simulink library "MATLAB_Function_lib"  (R2017b)
settings: Solver=VariableStepAuto  StartTime=0.0  StopTime=10.0  RelTol=1e-3
undefined symbols (not defined in the file or in its folder): Newton, Raphson
libraries: simulink x1
(part 2 of 3)

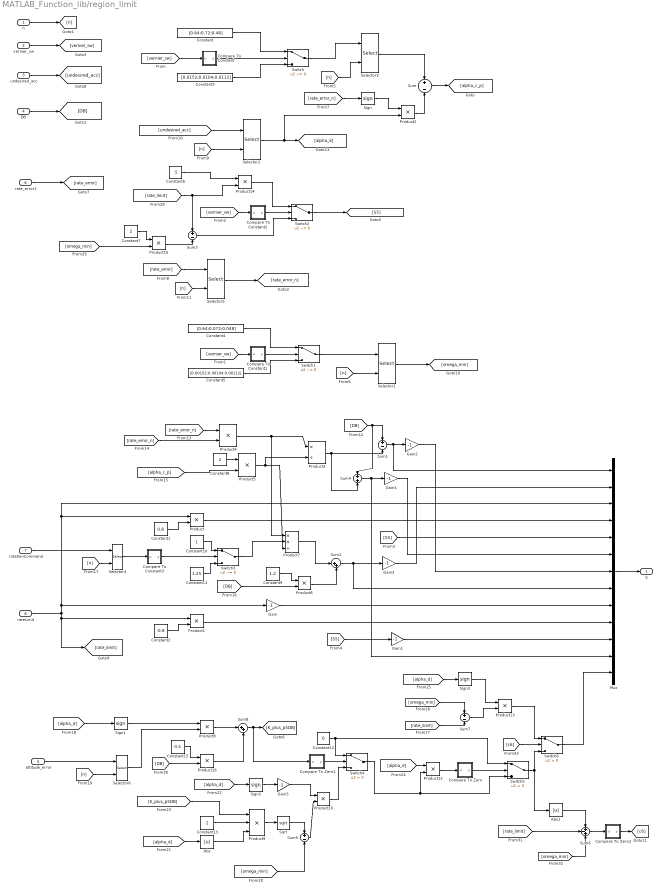
== system MATLAB_Function_lib/region_limit ==
  n : Inport
  vernier_sw : Inport  Port=2
  undesired_acc : Inport  Port=3
  DB : Inport  Port=4
  attitude_error : Inport  Port=5
  rate_error1 : Inport  Port=6
  rotationCommand : Inport  Port=7
  rateLimit : Inport  Port=8
  Abs : Abs
  Abs1 : Abs
  Compare To Constant : Subsystem  mask(Compare To Constant){relop===, const=1, OutDataTypeStr=boolean, ZeroCross=on}
      mask prompts: relop "Simulink:masks:Operator_MP"; const "Simulink:masks:ConstantValue_MP"; OutDataTypeStr "Simulink:masks:OutputDataType_MP"; ZeroCross "Simulink:masks:EnableZerocrossingDetection_MP"
      mask help: Simulink:masks:CompareToConstant_MD
      mask init: same as MATLAB_Function_lib/phase_plane/Compare To Constant
      mask TypeOptions relop: == | ~= | < | <= | >= | >
      mask TypeOptions OutDataTypeStr: Simulink:masks:uint8 | Simulink:masks:boolean
      mask Callback ZeroCross: sl('zeroCrossEnable', gcbh);
      mask Display: disp(str)
  Compare To Constant1 : Subsystem  mask(Compare To Constant){relop===, const=1, OutDataTypeStr=boolean, ZeroCross=on}
      mask prompts: relop "Simulink:masks:Operator_MP"; const "Simulink:masks:ConstantValue_MP"; OutDataTypeStr "Simulink:masks:OutputDataType_MP"; ZeroCross "Simulink:masks:EnableZerocrossingDetection_MP"
      mask help: Simulink:masks:CompareToConstant_MD
      mask init: same as MATLAB_Function_lib/phase_plane/Compare To Constant
      mask TypeOptions relop: == | ~= | < | <= | >= | >
      mask TypeOptions OutDataTypeStr: Simulink:masks:uint8 | Simulink:masks:boolean
      mask Callback ZeroCross: sl('zeroCrossEnable', gcbh);
      mask Display: disp(str)
  Compare To Constant2 : Subsystem  mask(Compare To Constant){relop===, const=0, OutDataTypeStr=boolean, ZeroCross=on}
      mask prompts: relop "Simulink:masks:Operator_MP"; const "Simulink:masks:ConstantValue_MP"; OutDataTypeStr "Simulink:masks:OutputDataType_MP"; ZeroCross "Simulink:masks:EnableZerocrossingDetection_MP"
      mask help: Simulink:masks:CompareToConstant_MD
      mask init: same as MATLAB_Function_lib/phase_plane/Compare To Constant
      mask TypeOptions relop: == | ~= | < | <= | >= | >
      mask TypeOptions OutDataTypeStr: Simulink:masks:uint8 | Simulink:masks:boolean
      mask Callback ZeroCross: sl('zeroCrossEnable', gcbh);
      mask Display: disp(str)
  Compare To Constant3 : Subsystem  mask(Compare To Constant){relop===, const=1, OutDataTypeStr=boolean, ZeroCross=on}
      mask prompts: relop "Simulink:masks:Operator_MP"; const "Simulink:masks:ConstantValue_MP"; OutDataTypeStr "Simulink:masks:OutputDataType_MP"; ZeroCross "Simulink:masks:EnableZerocrossingDetection_MP"
      mask help: Simulink:masks:CompareToConstant_MD
      mask init: same as MATLAB_Function_lib/phase_plane/Compare To Constant
      mask TypeOptions relop: == | ~= | < | <= | >= | >
      mask TypeOptions OutDataTypeStr: Simulink:masks:uint8 | Simulink:masks:boolean
      mask Callback ZeroCross: sl('zeroCrossEnable', gcbh);
      mask Display: disp(str)
  Compare To Zero : Subsystem  mask(Compare To Zero){relop=>, OutDataTypeStr=boolean, ZeroCross=on}
      mask prompts: relop "Simulink:masks:Operator_MP"; OutDataTypeStr "Simulink:masks:OutputDataType_MP"; ZeroCross "Simulink:masks:EnableZerocrossingDetection_MP"
      mask help: Simulink:masks:CompareToZero_MD
      mask init: same as MATLAB_Function_lib/affectation_region/Compare To Zero2
      mask TypeOptions relop: == | ~= | < | <= | >= | >
      mask TypeOptions OutDataTypeStr: Simulink:masks:uint8 | Simulink:masks:boolean
      mask Callback ZeroCross: sl('zeroCrossEnable', gcbh);
      mask Display: disp([relop,' 0'])
  Compare To Zero1 : Subsystem  mask(Compare To Zero){relop=<=, OutDataTypeStr=boolean, ZeroCross=on}
      mask prompts: relop "Simulink:masks:Operator_MP"; OutDataTypeStr "Simulink:masks:OutputDataType_MP"; ZeroCross "Simulink:masks:EnableZerocrossingDetection_MP"
      mask help: Simulink:masks:CompareToZero_MD
      mask init: same as MATLAB_Function_lib/affectation_region/Compare To Zero2
      mask TypeOptions relop: == | ~= | < | <= | >= | >
      mask TypeOptions OutDataTypeStr: Simulink:masks:uint8 | Simulink:masks:boolean
      mask Callback ZeroCross: sl('zeroCrossEnable', gcbh);
      mask Display: disp([relop,' 0'])
  Compare To Zero2 : Subsystem  mask(Compare To Zero){relop=>, OutDataTypeStr=boolean, ZeroCross=on}
      mask prompts: relop "Simulink:masks:Operator_MP"; OutDataTypeStr "Simulink:masks:OutputDataType_MP"; ZeroCross "Simulink:masks:EnableZerocrossingDetection_MP"
      mask help: Simulink:masks:CompareToZero_MD
      mask init: same as MATLAB_Function_lib/affectation_region/Compare To Zero2
      mask TypeOptions relop: == | ~= | < | <= | >= | >
      mask TypeOptions OutDataTypeStr: Simulink:masks:uint8 | Simulink:masks:boolean
      mask Callback ZeroCross: sl('zeroCrossEnable', gcbh);
      mask Display: disp([relop,' 0'])
  Constant : Constant  Value=[0.64;0.72;0.48]
  Constant1 : Constant  Value=0.8
  Constant10 : Constant
  Constant11 : Constant  Value=1.25
  Constant12 : Constant  Value=0
  Constant13 : Constant  Value=2
  Constant15 : Constant  Value=0.5
  Constant2 : Constant  Value=-0.8
  Constant3 : Constant  Value=[0.0152;0.0104;0.0112]
  Constant4 : Constant  Value=[0.64;0.072;0.048]
  Constant5 : Constant  Value=[0.00152;0.00104;0.00112]
  Constant6 : Constant  Value=.5
  Constant7 : Constant  Value=2
  Constant8 : Constant  Value=2
  Constant9 : Constant  Value=1.2
  Gain{,1..5} (6 alike) : Gain  Gain=-1
  Mux : Mux  Inputs=13
  Product{,1..2,6,8,10,12..16} (11 alike) : Product
  Product3 : Product  Inputs=*/
  Product4 : Product  Inputs=**
  Product5 : Product  Inputs=**
  Product7 : Product  Inputs=**/
  Product9 : Product  Inputs=3
  Selector{1..6} (6 alike) : Selector  InputPortWidth=3  IndexOptions=Index vector (port)  Indices=[1 3]  OutputSizes=1
  Sign{,1..3} (4 alike) : Signum
  Sqrt : Sqrt  SaturateOnIntegerOverflow=on
  Sum{,1,3,5,7} (5 alike) : Sum  Inputs=+-
  Sum2 : Sum  Inputs=|++
  Sum4 : Sum
  Sum6 : Sum  Inputs=+-+
  Sum8 : Sum  Inputs=|++
  Switch{,1..3} (4 alike) : Switch  Criteria=u2 ~= 0
  Switch4 : Switch  Criteria=u2 > Threshold
  Switch5 : Switch  Criteria=u2 > Threshold
  Switch6 : Switch  Criteria=u2 > Threshold
  S : Outport  PortDimensions=13
  wires:
  attitude_error/1 -> Selector6/1
  undesired_acc/1 -> [undesired_acc]
  vernier_sw/1 -> [vernier_sw]
  n/1 -> [n]
  DB/1 -> [DB]
  rate_error1/1 -> [rate_error]
  Mux/1 -> S/1
  Product/1 -> Mux/4
  Constant1/1 -> Product/2
  Product1/1 -> Mux/10
  rateLimit/1 -> Product1/1, [rate_limit], Mux/3, Product/1, Gain/1
  Constant2/1 -> Product1/2
  Gain/1 -> Mux/9
  [vernier_sw] -> Compare To Constant/1(u)
  Compare To Constant/1(y) -> Switch/2
  Constant/1 -> Switch/1
  Constant3/1 -> Switch/3
  Constant4/1 -> Switch1/1
  [vernier_sw] -> Compare To Constant1/1(u)
  Constant5/1 -> Switch1/3
  Compare To Constant1/1(y) -> Switch1/2
  Product14/1 -> Switch2/1
  [vernier_sw] -> Compare To Constant2/1(u)
  Sum3/1 -> Switch2/3
  Compare To Constant2/1(y) -> Switch2/2
  Switch2/1 -> [S5]
  [S5] -> Mux/5
  [S5] -> Gain1/1
  Gain1/1 -> Mux/11
  [n] -> Selector3/2
  Selector3/1 -> Sum/1
  Switch/1 -> Selector3/1
  Selector1/1 -> [omega_min]
  [n] -> Selector1/2
  Switch1/1 -> Selector1/1
  Selector2/1 -> Product2/2, [alpha_d]
  [n] -> Selector2/2
  [undesired_acc] -> Selector2/1
  Product2/1 -> Sum/2
  Sum/1 -> [alpha_c_p]
  [rate_error_n] -> Sign/1
  Sign/1 -> Product2/1
  [rate_error] -> Selector5/1
  Selector5/1 -> [rate_error_n]
  [n] -> Selector5/2
  [DB] -> Sum4/1, Sum1/1
  Product3/1 -> Sum4/2, Sum1/2
  [rate_error_n] -> Product4/1
  [rate_error_n] -> Product4/2
  Product4/1 -> Product7/1, Product3/1
  Product5/1 -> Product7/3, Product3/2
  Constant8/1 -> Product5/1
  [alpha_c_p] -> Product5/2
  Sum1/1 -> Mux/1, Gain2/1
  Gain2/1 -> Mux/7
  Product6/1 -> Sum2/2
  Constant9/1 -> Product6/1
  [DB] -> Product6/2
  Sum2/1 -> Mux/8, Gain3/1
  Gain3/1 -> Mux/2
  Product7/1 -> Sum2/1
  Switch3/1 -> Product7/2
  Constant10/1 -> Switch3/1
  Constant11/1 -> Switch3/3
  [n] -> Selector4/2
  rotationCommand/1 -> Selector4/1
  Compare To Constant3/1(y) -> Switch3/2
  Selector4/1 -> Compare To Constant3/1(u)
  Sum4/1 -> Gain4/1, Mux/12
  Gain4/1 -> Mux/6
  Sign1/1 -> Product8/1
  [alpha_d] -> Sign1/1
  Selector6/1 -> Product8/2
  [n] -> Selector6/2
  Product8/1 -> Sum8/1
  Constant12/1 -> Switch5/1, Switch4/1
  [omega_min] -> Sum5/2
  [alpha_d] -> Abs/1
  Abs/1 -> Product9/3
  Constant13/1 -> Product9/2
  Product9/1 -> Sqrt/1
  Sqrt/1 -> Sum5/1
  Sum5/1 -> Product10/2
  [alpha_d] -> Sign2/1
  Sign2/1 -> Gain5/1
  Gain5/1 -> Product10/1
  Product10/1 -> Switch4/3
  [K_plus_p5DB] -> Product9/1
  Product12/1 -> Compare To Zero/1(u)
  Compare To Zero/1(y) -> Switch5/2
  [alpha_d] -> Product12/1
  Switch4/1 -> Switch5/3, Product12/2
  [alpha_d] -> Sign3/1
  Sign3/1 -> Product13/1
  Product13/1 -> Switch6/1
  Switch5/1 -> Abs1/1, Switch6/3
  [omega_min] -> Sum7/1
  [rate_limit] -> Sum7/2
  Sum7/1 -> Product13/2
  Switch6/1 -> Mux/13
  Constant6/1 -> Product14/1
  [rate_limit] -> Sum3/1, Product14/2
  Product15/1 -> Sum3/2
  Constant7/1 -> Product15/1
  [omega_min] -> Product15/2
  Constant15/1 -> Product16/1
  [DB] -> Product16/2
  Product16/1 -> Sum8/2
  Sum8/1 -> Compare To Zero1/1(u), [K_plus_p5DB]
  Compare To Zero1/1(y) -> Switch4/2
  Compare To Zero2/1(y) -> [c6]
  Sum6/1 -> Compare To Zero2/1(u)
  Abs1/1 -> Sum6/1
  [rate_limit] -> Sum6/2
  [omega_min] -> Sum6/3
  [c6] -> Switch6/2

== system MATLAB_Function_lib/vernier_jet_logic ==
  Constant : Constant  Value=zeros(6,1)
  Out1 : Outport
  wires:
  Constant/1 -> Out1/1

== system MATLAB_Function_lib/Direction Cosine Matrix to Quaternions/Negative Trace ==
  DCM : Inport
  Action Port : ActionPort  PropagateVarSize=During execution  ActionType=else
  Find Maximum Diagonal Value : If  NumInputs=3  IfExpression=((u2 > u1) & (u2 > u3))  ElseIfExpressions=u3 > u1
  Maximum Value at DCM(1,1) : Subsystem
  Maximum Value at DCM(2,2) : Subsystem
  Maximum Value at DCM(3,3) : Subsystem
  Merge1 : Merge  Inputs=3
  diag(DCM) : Subsystem
  qw qx qy qz : Outport
  wires:
  Find Maximum Diagonal Value/2 -> Maximum Value at DCM(3,3)/Action
  DCM/1 -> diag(DCM)/1(DCM), Maximum Value at DCM(2,2)/1(DCM), Maximum Value at DCM(1,1)/1(DCM), Maximum Value at DCM(3,3)/1(DCM)
  diag(DCM)/1(u(1)) -> Find Maximum Diagonal Value/1
  Merge1/1 -> qw qx qy qz/1
  Maximum Value at DCM(1,1)/1(qw qx qy qz) -> Merge1/3
  diag(DCM)/3(u(9)) -> Find Maximum Diagonal Value/3
  Maximum Value at DCM(2,2)/1(qw qx qy qz) -> Merge1/1
  Find Maximum Diagonal Value/3 -> Maximum Value at DCM(1,1)/Action
  Maximum Value at DCM(3,3)/1(qw qx qy qz) -> Merge1/2
  diag(DCM)/2(u(5)) -> Find Maximum Diagonal Value/2
  Find Maximum Diagonal Value/1 -> Maximum Value at DCM(2,2)/Action

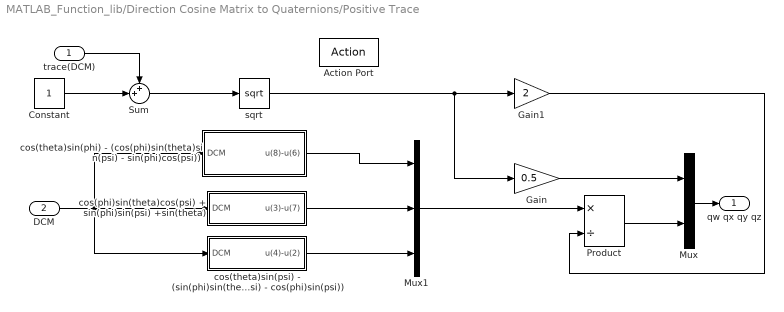
== system MATLAB_Function_lib/Direction Cosine Matrix to Quaternions/Positive Trace ==
  trace(DCM) : Inport
  DCM : Inport  Port=2
  Action Port : ActionPort  PropagateVarSize=During execution  ActionType=then
  Constant : Constant  OutDataTypeStr=Inherit: Inherit via back propagation
  Gain : Gain  Gain=0.5  OutDataTypeStr=Inherit: Inherit via back propagation  SaturateOnIntegerOverflow=on  ParamDataTypeStr=Inherit: Same as input
  Gain1 : Gain  Gain=2  OutDataTypeStr=Inherit: Inherit via back propagation  SaturateOnIntegerOverflow=on  ParamDataTypeStr=Inherit: Same as input
  Mux : Mux  Inputs=2
  Mux1 : Mux  Inputs=3
  Product : Product  Inputs=*/  SaturateOnIntegerOverflow=on  InputSameDT=on  OutDataTypeStr=Inherit: Same as first input
  Sum : Sum  Inputs=++|  SaturateOnIntegerOverflow=on  InputSameDT=on  OutDataTypeStr=Inherit: Same as first input
  cos(phi)sin(theta)cos(psi) + sin(phi)sin(psi) +sin(theta) : Subsystem
  cos(theta)sin(phi) - (cos(phi)sin(theta)sin(psi) - sin(phi)cos(psi)) : Subsystem
  cos(theta)sin(psi) - (sin(phi)sin(theta)cos(psi) - cos(phi)sin(psi)) : Subsystem
  sqrt : Sqrt  AlgorithmType=Newton-Raphson  SaturateOnIntegerOverflow=on
  qw qx qy qz : Outport
  wires:
  sqrt/1 -> Gain/1, Gain1/1
  trace(DCM)/1 -> Sum/1
  Mux1/1 -> Product/1
  Constant/1 -> Sum/2
  Sum/1 -> sqrt/1
  Gain1/1 -> Product/2
  Gain/1 -> Mux/1
  Mux/1 -> qw qx qy qz/1
  Product/1 -> Mux/2
  cos(phi)sin(theta)cos(psi) + sin(phi)sin(psi) +sin(theta)/1(u(3)-u(7)) -> Mux1/2
  cos(theta)sin(psi) - (sin(phi)sin(theta)cos(psi) - cos(phi)sin(psi))/1(u(4)-u(2)) -> Mux1/3
  cos(theta)sin(phi) - (cos(phi)sin(theta)sin(psi) - sin(phi)cos(psi))/1(u(8)-u(6)) -> Mux1/1
  DCM/1 -> cos(theta)sin(phi) - (cos(phi)sin(theta)sin(psi) - sin(phi)cos(psi))/1(DCM), cos(phi)sin(theta)cos(psi) + sin(phi)sin(psi) +sin(theta)/1(DCM), cos(theta)sin(psi) - (sin(phi)sin(theta)cos(psi) - cos(phi)sin(psi))/1(DCM)

== system MATLAB_Function_lib/Direction Cosine Matrix to Quaternions/trace(DCM) ==
  DCM : Inport
  Add : Sum  Inputs=+
  Selector : Selector  InputPortWidth=9  IndexOptions=Index vector (dialog)  Indices=[1 5 9]  OutputSizes=1
  trace(DCM) : Outport
  wires:
  DCM/1 -> Selector/1
  Selector/1 -> Add/1
  Add/1 -> trace(DCM)/1

== system MATLAB_Function_lib/Quaternion Multiplication/q0 ==
  q : Inport
  r : Inport  Port=2
  Demux : Demux
  Demux1 : Demux
  Product{,1..3} (4 alike) : Product  RndMeth=Zero
  Sum : Sum  Inputs=+---
  q0 : Outport
  wires:
  Product2/1 -> Sum/3
  Sum/1 -> q0/1
  Product3/1 -> Sum/4
  Product1/1 -> Sum/2
  Product/1 -> Sum/1
  Demux/4 -> Product3/1
  Demux1/4 -> Product3/2
  Demux1/3 -> Product2/2
  Demux/3 -> Product2/1
  Demux1/2 -> Product1/2
  Demux/2 -> Product1/1
  Demux1/1 -> Product/2
  Demux/1 -> Product/1
  r/1 -> Demux1/1
  q/1 -> Demux/1

== system MATLAB_Function_lib/Quaternion Multiplication/q1 ==
  q : Inport
  r : Inport  Port=2
  Demux : Demux
  Demux1 : Demux
  Product{,1..3} (4 alike) : Product  RndMeth=Zero
  Sum : Sum  Inputs=+++-
  q1 : Outport
  wires:
  Demux1/3 -> Product3/2
  Demux1/4 -> Product2/2
  Demux1/1 -> Product1/2
  Demux1/2 -> Product/2
  q/1 -> Demux/1
  r/1 -> Demux1/1
  Demux/1 -> Product/1
  Demux/2 -> Product1/1
  Demux/3 -> Product2/1
  Demux/4 -> Product3/1
  Product/1 -> Sum/1
  Product1/1 -> Sum/2
  Product3/1 -> Sum/4
  Sum/1 -> q1/1
  Product2/1 -> Sum/3

== system MATLAB_Function_lib/Quaternion Multiplication/q2 ==
  q : Inport
  r : Inport  Port=2
  Demux : Demux
  Demux1 : Demux
  Product{,1..3} (4 alike) : Product  RndMeth=Zero
  Sum : Sum  Inputs=+-++
  q2 : Outport
  wires:
  Demux1/2 -> Product3/2
  Demux1/1 -> Product2/2
  Demux1/4 -> Product1/2
  Demux1/3 -> Product/2
  Product2/1 -> Sum/3
  Sum/1 -> q2/1
  Product3/1 -> Sum/4
  Product1/1 -> Sum/2
  Product/1 -> Sum/1
  Demux/4 -> Product3/1
  Demux/3 -> Product2/1
  Demux/2 -> Product1/1
  Demux/1 -> Product/1
  r/1 -> Demux1/1
  q/1 -> Demux/1

== system MATLAB_Function_lib/Quaternion Multiplication/q3 ==
  q : Inport
  r : Inport  Port=2
  Demux : Demux
  Demux1 : Demux
  Product{,1..3} (4 alike) : Product  RndMeth=Zero
  Sum : Sum  Inputs=++-+
  q3 : Outport
  wires:
  Demux1/4 -> Product/2
  Demux1/3 -> Product1/2
  Demux1/1 -> Product3/2
  Demux1/2 -> Product2/2
  q/1 -> Demux/1
  r/1 -> Demux1/1
  Demux/1 -> Product/1
  Demux/2 -> Product1/1
  Demux/3 -> Product2/1
  Demux/4 -> Product3/1
  Product/1 -> Sum/1
  Product1/1 -> Sum/2
  Product3/1 -> Sum/4
  Sum/1 -> q3/1
  Product2/1 -> Sum/3

== system MATLAB_Function_lib/Rotation Angles to Direction Cosine Matrix/Create 3x3 Matrix ==
  M11 : Inport  PortDimensions=1
  M12 : Inport  Port=2  PortDimensions=1
  M13 : Inport  Port=3  PortDimensions=1
  M21 : Inport  Port=4  PortDimensions=1
  M22 : Inport  Port=5  PortDimensions=1
  M23 : Inport  Port=6  PortDimensions=1
  M31 : Inport  Port=7  PortDimensions=1
  M32 : Inport  Port=8  PortDimensions=1
  M33 : Inport  Port=9  PortDimensions=1
  Reshape (9) to [3x3] column-major : Reshape  OutputDimensionality=Customize  OutputDimensions=[3,3]
  Vector Concatenate : Concatenate  NumInputs=9
  Matrix : Outport  PortDimensions=[3 3]
  wires:
  M33/1 -> Vector Concatenate/9
  M23/1 -> Vector Concatenate/8
  M13/1 -> Vector Concatenate/7
  M32/1 -> Vector Concatenate/6
  Reshape (9) to [3x3] column-major/1 -> Matrix/1
  M22/1 -> Vector Concatenate/5
  M12/1 -> Vector Concatenate/4
  M31/1 -> Vector Concatenate/3
  M21/1 -> Vector Concatenate/2
  M11/1 -> Vector Concatenate/1
  Vector Concatenate/1 -> Reshape (9) to [3x3] column-major/1

== system MATLAB_Function_lib/affectation_region/Compare To Zero2 ==
  u : Inport
  Compare : RelationalOperator  Operator=>  OutDataTypeStr=boolean  RndMeth=Nearest  InputSameDT=on
  Constant : Constant  DisableCoverage=on  Value=0  OutDataTypeStr=Inherit: Inherit via back propagation  PreserveConstantTs=on
  y : Outport
  wires:
  Constant/1 -> Compare/2
  u/1 -> Compare/1
  Compare/1 -> y/1

== system MATLAB_Function_lib/affectation_region/Compare To Zero20 ==
  u : Inport
  Compare : RelationalOperator  OutDataTypeStr=boolean  RndMeth=Nearest  InputSameDT=on
  Constant : Constant  DisableCoverage=on  Value=0  OutDataTypeStr=Inherit: Inherit via back propagation  PreserveConstantTs=on
  y : Outport
  wires:
  Constant/1 -> Compare/2
  u/1 -> Compare/1
  Compare/1 -> y/1

== system MATLAB_Function_lib/affectation_region/Compare To Zero23 ==
  u : Inport
  Compare : RelationalOperator  OutDataTypeStr=boolean  RndMeth=Nearest  InputSameDT=on
  Constant : Constant  DisableCoverage=on  Value=0  OutDataTypeStr=Inherit: Inherit via back propagation  PreserveConstantTs=on
  y : Outport
  wires:
  Constant/1 -> Compare/2
  u/1 -> Compare/1
  Compare/1 -> y/1

== system MATLAB_Function_lib/affectation_region/Compare To Zero26 ==
  u : Inport
  Compare : RelationalOperator  Operator=<  OutDataTypeStr=boolean  RndMeth=Nearest  InputSameDT=on
  Constant : Constant  DisableCoverage=on  Value=0  OutDataTypeStr=Inherit: Inherit via back propagation  PreserveConstantTs=on
  y : Outport
  wires:
  Constant/1 -> Compare/2
  u/1 -> Compare/1
  Compare/1 -> y/1

== system MATLAB_Function_lib/affectation_region/Compare To Zero39 ==
  u : Inport
  Compare : RelationalOperator  Operator=<=  OutDataTypeStr=boolean  RndMeth=Nearest  InputSameDT=on
  Constant : Constant  DisableCoverage=on  Value=0  OutDataTypeStr=Inherit: Inherit via back propagation  PreserveConstantTs=on
  y : Outport
  wires:
  Constant/1 -> Compare/2
  u/1 -> Compare/1
  Compare/1 -> y/1

== system MATLAB_Function_lib/affectation_region/Compare To Zero42 ==
  u : Inport
  Compare : RelationalOperator  Operator=>  OutDataTypeStr=boolean  RndMeth=Nearest  InputSameDT=on
  Constant : Constant  DisableCoverage=on  Value=0  OutDataTypeStr=Inherit: Inherit via back propagation  PreserveConstantTs=on
  y : Outport
  wires:
  Constant/1 -> Compare/2
  u/1 -> Compare/1
  Compare/1 -> y/1

== system MATLAB_Function_lib/affectation_region/Compare To Zero7 ==
  u : Inport
  Compare : RelationalOperator  Operator=<=  OutDataTypeStr=boolean  RndMeth=Nearest  InputSameDT=on
  Constant : Constant  DisableCoverage=on  Value=0  OutDataTypeStr=Inherit: Inherit via back propagation  PreserveConstantTs=on
  y : Outport
  wires:
  Constant/1 -> Compare/2
  u/1 -> Compare/1
  Compare/1 -> y/1

== system MATLAB_Function_lib/get_delta_omega/For Iterator Subsystem ==
  JetCommand : Inport
  matrix_delta_omega_jet : Inport  Port=2
  Compare To Constant : Subsystem  mask(Compare To Constant){relop===, const=1, OutDataTypeStr=boolean, ZeroCross=on}
      mask prompts: relop "Simulink:masks:Operator_MP"; const "Simulink:masks:ConstantValue_MP"; OutDataTypeStr "Simulink:masks:OutputDataType_MP"; ZeroCross "Simulink:masks:EnableZerocrossingDetection_MP"
      mask help: Simulink:masks:CompareToConstant_MD
      mask init: same as MATLAB_Function_lib/phase_plane/Compare To Constant
      mask TypeOptions relop: == | ~= | < | <= | >= | >
      mask TypeOptions OutDataTypeStr: Simulink:masks:uint8 | Simulink:masks:boolean
      mask Callback ZeroCross: sl('zeroCrossEnable', gcbh);
      mask Display: disp(str)
  For Iterator : ForIterator  ResetStates=reset  IterationLimit=11
  Reshape : Reshape  OutputDimensionality=Column vector (2-D)
  Selector1 : Selector  InputPortWidth=11  IndexOptions=Index vector (port)  Indices=[1 3]  OutputSizes=1
  Selector2 : Selector  NumberOfDimensions=2  InputPortWidth=3  IndexOptions=Index vector (port),Select all  Indices=[1 3],1  OutputSizes=1,1
  Sum : Sum  Inputs=|++
  Switch : Switch  Criteria=u2 ~= 0
  Unit Delay : UnitDelay  InitialCondition=[0; 0; 0]  SampleTime=-1
  Out1 : Outport
  wires:
  matrix_delta_omega_jet/1 -> Selector2/1
  For Iterator/1 -> Selector1/2, Selector2/2
  JetCommand/1 -> Selector1/1
  Selector1/1 -> Compare To Constant/1(u)
  Compare To Constant/1(y) -> Switch/2
  Sum/1 -> Switch/1
  Selector2/1 -> Reshape/1
  Switch/1 -> Unit Delay/1, Out1/1
  Unit Delay/1 -> Sum/2, Switch/3
  Reshape/1 -> Sum/1

== system MATLAB_Function_lib/phase_plane/Compare To Constant ==
  u : Inport
  Compare : RelationalOperator  Operator===  OutDataTypeStr=boolean  RndMeth=Nearest  InputSameDT=on
  Constant : Constant  DisableCoverage=on  Value=const  OutDataTypeStr=Inherit: Inherit via back propagation
  y : Outport
  wires:
  u/1 -> Compare/1
  Constant/1 -> Compare/2
  Compare/1 -> y/1

== system MATLAB_Function_lib/phase_plane/Compare To Constant1 ==
  u : Inport
  Compare : RelationalOperator  Operator===  OutDataTypeStr=boolean  RndMeth=Nearest  InputSameDT=on
  Constant : Constant  DisableCoverage=on  Value=const  OutDataTypeStr=Inherit: Inherit via back propagation
  y : Outport
  wires:
  u/1 -> Compare/1
  Constant/1 -> Compare/2
  Compare/1 -> y/1

== system MATLAB_Function_lib/phase_plane/Compare To Constant2 ==
  u : Inport
  Compare : RelationalOperator  Operator===  OutDataTypeStr=boolean  RndMeth=Nearest  InputSameDT=on
  Constant : Constant  DisableCoverage=on  Value=const  OutDataTypeStr=Inherit: Inherit via back propagation
  y : Outport
  wires:
  u/1 -> Compare/1
  Constant/1 -> Compare/2
  Compare/1 -> y/1

== system MATLAB_Function_lib/phase_plane/Compare To Constant3 ==
  u : Inport
  Compare : RelationalOperator  Operator===  OutDataTypeStr=boolean  RndMeth=Nearest  InputSameDT=on
  Constant : Constant  DisableCoverage=on  Value=const  OutDataTypeStr=Inherit: Inherit via back propagation
  y : Outport
  wires:
  u/1 -> Compare/1
  Constant/1 -> Compare/2
  Compare/1 -> y/1

== system MATLAB_Function_lib/phase_plane/If Action Subsystem ==
  Action Port : ActionPort
  Constant : Constant  Value=-1
  Out1 : Outport
  wires:
  Constant/1 -> Out1/1

== system MATLAB_Function_lib/phase_plane/If Action Subsystem1 ==
  Action Port : ActionPort
  Constant : Constant
  Out1 : Outport
  wires:
  Constant/1 -> Out1/1

== system MATLAB_Function_lib/phase_plane/If Action Subsystem2 ==
  Action Port : ActionPort
  Constant : Constant  Value=0
  Out1 : Outport
  wires:
  Constant/1 -> Out1/1

== system MATLAB_Function_lib/phase_plane/If Action Subsystem3 ==
  we : Inport
  rateLimit : Inport  Port=2
  Action Port : ActionPort
  Constant : Constant  Value=3.2
  Constant1 : Constant  Value=4
  Product : Product  Inputs=**/
  Sum : Sum  Inputs=+-
  Out1 : Outport
  wires:
  Sum/1 -> Out1/1
  Constant/1 -> Sum/1
  Product/1 -> Sum/2
  rateLimit/1 -> Product/3
  we/1 -> Product/2
  Constant1/1 -> Product/1

== system MATLAB_Function_lib/phase_plane/If Action Subsystem4 ==
  we : Inport
  rateLimit : Inport  Port=2
  Action Port : ActionPort
  Constant : Constant  Value=3.2
  Constant1 : Constant  Value=4
  Product : Product  Inputs=**/
  Sum : Sum  Inputs=+-
  Out1 : Outport
  wires:
  Product/1 -> Sum/2
  Constant/1 -> Sum/1
  Constant1/1 -> Product/1
  we/1 -> Product/2
  rateLimit/1 -> Product/3
  Sum/1 -> Out1/1

== system MATLAB_Function_lib/phase_plane/If Action Subsystem5 ==
  forceFire_n : Inport
  S13 : Inport  Port=2
  we : Inport  Port=3
  rateLimit : Inport  Port=4
  Action Port : ActionPort
  Constant : Constant  Value=-1  SampleTime=-1
  Constant1 : Constant  Value=0.8
  Product : Product  Inputs=**/
  Sum : Sum  Inputs=+-
  Sum1 : Sum  Inputs=+-
  Switch : Switch  Criteria=u2 ~= 0
  Out1 : Outport
  wires:
  Switch/1 -> Out1/1
  forceFire_n/1 -> Switch/2
  Constant/1 -> Switch/1
  Product/1 -> Switch/3
  Constant1/1 -> Product/1
  S13/1 -> Sum1/2, Sum/1
  we/1 -> Sum/2
  Sum1/1 -> Product/3
  Sum/1 -> Product/2
  rateLimit/1 -> Sum1/1

== system MATLAB_Function_lib/phase_plane/If Action Subsystem6 ==
  forceFire_n : Inport
  S13 : Inport  Port=2
  we : Inport  Port=3
  rateLimit : Inport  Port=4
  Action Port : ActionPort
  Constant : Constant  SampleTime=-1
  Constant1 : Constant  Value=0.8
  Product : Product  Inputs=**/
  Sum : Sum  Inputs=+-
  Sum1 : Sum
  Switch : Switch  Criteria=u2 ~= 0
  Out1 : Outport
  wires:
  Switch/1 -> Out1/1
  we/1 -> Sum/2
  Constant1/1 -> Product/1
  S13/1 -> Sum1/2, Sum/1
  Sum1/1 -> Product/3
  Product/1 -> Switch/3
  forceFire_n/1 -> Switch/2
  Constant/1 -> Switch/1
  Sum/1 -> Product/2
  rateLimit/1 -> Sum1/1

== system MATLAB_Function_lib/phase_plane/If Action Subsystem7 ==
  S13 : Inport
  we : Inport  Port=2
  rateLimit : Inport  Port=3
  Action Port : ActionPort
  Constant1 : Constant  Value=0.8
  Product : Product  Inputs=3
  Product1 : Product
  Sign : Signum
  Sum : Sum  Inputs=+-
  Sum1 : Sum  Inputs=+-
  Out1 : Outport
  wires:
  we/1 -> Sign/1, Sum/2
  Sum1/1 -> Product/3
  rateLimit/1 -> Sum1/1
  Product/1 -> Out1/1
  Sum/1 -> Product/2
  Constant1/1 -> Product/1
  S13/1 -> Product1/1, Sum/1
  Product1/1 -> Sum1/2
  Sign/1 -> Product1/2

== system MATLAB_Function_lib/phase_plane/If Action Subsystem8 ==
  Action Port : ActionPort  ActionType=else
  Constant3 : Constant  Value=-100
  Out1 : Outport
  wires:
  Constant3/1 -> Out1/1

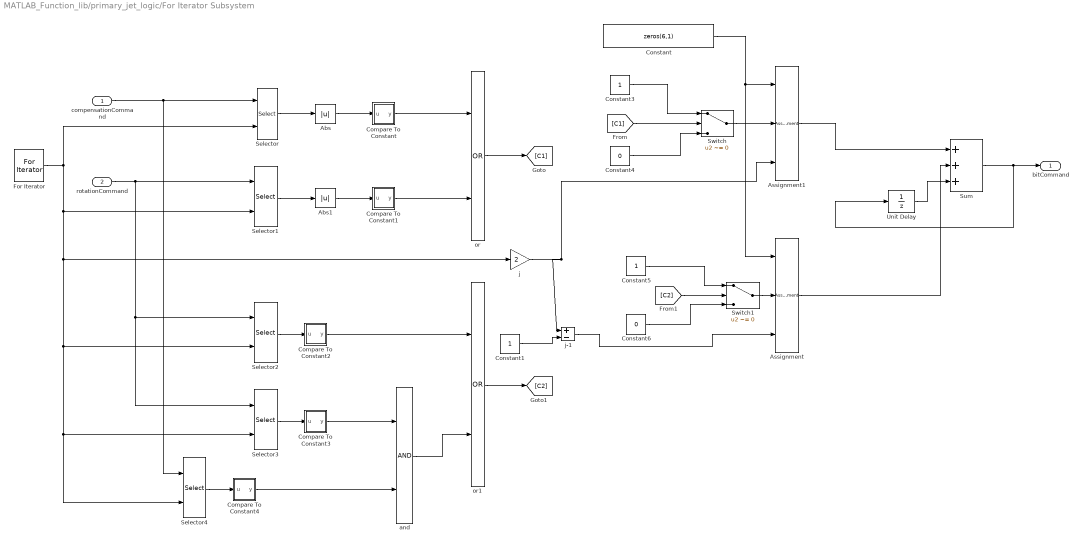
== system MATLAB_Function_lib/primary_jet_logic/For Iterator Subsystem ==
  compensationCommand : Inport
  rotationCommand : Inport  Port=2
  Abs : Abs
  Abs1 : Abs
  Assignment : Assignment  DiagnosticForDimensions=Warning  IndexOptions=Index vector (port)  Indices=1  OutputSizes=1
  Assignment1 : Assignment  DiagnosticForDimensions=Warning  IndexOptions=Index vector (port)  Indices=1  OutputSizes=1
  Compare To Constant : Subsystem  mask(Compare To Constant){relop===, const=1, OutDataTypeStr=boolean, ZeroCross=on}
      mask prompts: relop "Simulink:masks:Operator_MP"; const "Simulink:masks:ConstantValue_MP"; OutDataTypeStr "Simulink:masks:OutputDataType_MP"; ZeroCross "Simulink:masks:EnableZerocrossingDetection_MP"
      mask help: Simulink:masks:CompareToConstant_MD
      mask init: same as MATLAB_Function_lib/phase_plane/Compare To Constant
      mask TypeOptions relop: == | ~= | < | <= | >= | >
      mask TypeOptions OutDataTypeStr: Simulink:masks:uint8 | Simulink:masks:boolean
      mask Callback ZeroCross: sl('zeroCrossEnable', gcbh);
      mask Display: disp(str)
  Compare To Constant1 : Subsystem  mask(Compare To Constant){relop===, const=1, OutDataTypeStr=boolean, ZeroCross=on}
      mask prompts: relop "Simulink:masks:Operator_MP"; const "Simulink:masks:ConstantValue_MP"; OutDataTypeStr "Simulink:masks:OutputDataType_MP"; ZeroCross "Simulink:masks:EnableZerocrossingDetection_MP"
      mask help: Simulink:masks:CompareToConstant_MD
      mask init: same as MATLAB_Function_lib/phase_plane/Compare To Constant
      mask TypeOptions relop: == | ~= | < | <= | >= | >
      mask TypeOptions OutDataTypeStr: Simulink:masks:uint8 | Simulink:masks:boolean
      mask Callback ZeroCross: sl('zeroCrossEnable', gcbh);
      mask Display: disp(str)
  Compare To Constant2 : Subsystem  mask(Compare To Constant){relop===, const=-1, OutDataTypeStr=boolean, ZeroCross=on}
      mask prompts: relop "Simulink:masks:Operator_MP"; const "Simulink:masks:ConstantValue_MP"; OutDataTypeStr "Simulink:masks:OutputDataType_MP"; ZeroCross "Simulink:masks:EnableZerocrossingDetection_MP"
      mask help: Simulink:masks:CompareToConstant_MD
      mask init: same as MATLAB_Function_lib/phase_plane/Compare To Constant
      mask TypeOptions relop: == | ~= | < | <= | >= | >
      mask TypeOptions OutDataTypeStr: Simulink:masks:uint8 | Simulink:masks:boolean
      mask Callback ZeroCross: sl('zeroCrossEnable', gcbh);
      mask Display: disp(str)
  Compare To Constant3 : Subsystem  mask(Compare To Constant){relop=~=, const=1, OutDataTypeStr=boolean, ZeroCross=on}
      mask prompts: relop "Simulink:masks:Operator_MP"; const "Simulink:masks:ConstantValue_MP"; OutDataTypeStr "Simulink:masks:OutputDataType_MP"; ZeroCross "Simulink:masks:EnableZerocrossingDetection_MP"
      mask help: Simulink:masks:CompareToConstant_MD
      mask init: same as MATLAB_Function_lib/phase_plane/Compare To Constant
      mask TypeOptions relop: == | ~= | < | <= | >= | >
      mask TypeOptions OutDataTypeStr: Simulink:masks:uint8 | Simulink:masks:boolean
      mask Callback ZeroCross: sl('zeroCrossEnable', gcbh);
      mask Display: disp(str)
  Compare To Constant4 : Subsystem  mask(Compare To Constant){relop===, const=-1, OutDataTypeStr=boolean, ZeroCross=on}
      mask prompts: relop "Simulink:masks:Operator_MP"; const "Simulink:masks:ConstantValue_MP"; OutDataTypeStr "Simulink:masks:OutputDataType_MP"; ZeroCross "Simulink:masks:EnableZerocrossingDetection_MP"
      mask help: Simulink:masks:CompareToConstant_MD
      mask init: same as MATLAB_Function_lib/phase_plane/Compare To Constant
      mask TypeOptions relop: == | ~= | < | <= | >= | >
      mask TypeOptions OutDataTypeStr: Simulink:masks:uint8 | Simulink:masks:boolean
      mask Callback ZeroCross: sl('zeroCrossEnable', gcbh);
      mask Display: disp(str)
  Constant : Constant  Value=zeros(6,1)
  Constant1 : Constant
  Constant3 : Constant
  Constant4 : Constant  Value=0
  Constant5 : Constant
  Constant6 : Constant  Value=0
  For Iterator : ForIterator  ResetStates=reset  IterationLimit=3
  Selector{,1..4} (5 alike) : Selector  InputPortWidth=3  IndexOptions=Index vector (port)  Indices=[2]  OutputSizes=1
  Sum : Sum  Inputs=3
  Switch : Switch  Criteria=u2 ~= 0
  Switch1 : Switch  Criteria=u2 ~= 0
  Unit Delay : UnitDelay  InitialCondition=[0;0;0;0;0;0]  SampleTime=-1
  and : Logic  AllPortsSameDT=off  OutDataTypeStr=boolean
  j : Gain  Gain=2  OutDataTypeStr=int32
  j-1 : Sum  Inputs=+-
  or : Logic  Operator=OR  AllPortsSameDT=off  OutDataTypeStr=boolean
  or1 : Logic  Operator=OR  AllPortsSameDT=off  OutDataTypeStr=boolean
  bitCommand : Outport
  wires:
  Selector/1 -> Abs/1
  Abs/1 -> Compare To Constant/1(u)
  Compare To Constant/1(y) -> or/1
  Selector1/1 -> Abs1/1
  Abs1/1 -> Compare To Constant1/1(u)
  Compare To Constant1/1(y) -> or/2
  Selector2/1 -> Compare To Constant2/1(u)
  Compare To Constant2/1(y) -> or1/1
  and/1 -> or1/2
  rotationCommand/1 -> Selector1/1, Selector2/1, Selector3/1
  Selector3/1 -> Compare To Constant3/1(u)
  Compare To Constant3/1(y) -> and/1
  compensationCommand/1 -> Selector4/1, Selector/1
  Selector4/1 -> Compare To Constant4/1(u)
  Compare To Constant4/1(y) -> and/2
  For Iterator/1 -> Selector4/2, Selector3/2, Selector2/2, j/1, Selector1/2, Selector/2
  Assignment/1 -> Sum/2
  Constant1/1 -> j-1/2
  j-1/1 -> Assignment/3
  j/1 -> Assignment1/3, j-1/1
  Assignment1/1 -> Sum/1
  or/1 -> [C1]
  or1/1 -> [C2]
  [C1] -> Switch/2
  Switch/1 -> Assignment1/2
  Constant3/1 -> Switch/1
  Constant4/1 -> Switch/3
  Constant5/1 -> Switch1/1
  Constant6/1 -> Switch1/3
  [C2] -> Switch1/2
  Switch1/1 -> Assignment/2
  Constant/1 -> Assignment/1, Assignment1/1
  Sum/1 -> Unit Delay/1, bitCommand/1
  Unit Delay/1 -> Sum/3

== system MATLAB_Function_lib/region_limit/Compare To Constant ==
  u : Inport
  Compare : RelationalOperator  Operator===  OutDataTypeStr=boolean  RndMeth=Nearest  InputSameDT=on
  Constant : Constant  DisableCoverage=on  Value=const  OutDataTypeStr=Inherit: Inherit via back propagation
  y : Outport
  wires:
  u/1 -> Compare/1
  Constant/1 -> Compare/2
  Compare/1 -> y/1

== system MATLAB_Function_lib/region_limit/Compare To Constant1 ==
  u : Inport
  Compare : RelationalOperator  Operator===  OutDataTypeStr=boolean  RndMeth=Nearest  InputSameDT=on
  Constant : Constant  DisableCoverage=on  Value=const  OutDataTypeStr=Inherit: Inherit via back propagation
  y : Outport
  wires:
  u/1 -> Compare/1
  Constant/1 -> Compare/2
  Compare/1 -> y/1

== system MATLAB_Function_lib/region_limit/Compare To Constant2 ==
  u : Inport
  Compare : RelationalOperator  Operator===  OutDataTypeStr=boolean  RndMeth=Nearest  InputSameDT=on
  Constant : Constant  DisableCoverage=on  Value=const  OutDataTypeStr=Inherit: Inherit via back propagation
  y : Outport
  wires:
  u/1 -> Compare/1
  Constant/1 -> Compare/2
  Compare/1 -> y/1

== system MATLAB_Function_lib/region_limit/Compare To Constant3 ==
  u : Inport
  Compare : RelationalOperator  Operator===  OutDataTypeStr=boolean  RndMeth=Nearest  InputSameDT=on
  Constant : Constant  DisableCoverage=on  Value=const  OutDataTypeStr=Inherit: Inherit via back propagation
  y : Outport
  wires:
  u/1 -> Compare/1
  Constant/1 -> Compare/2
  Compare/1 -> y/1

== system MATLAB_Function_lib/region_limit/Compare To Zero ==
  u : Inport
  Compare : RelationalOperator  Operator=>  OutDataTypeStr=boolean  RndMeth=Nearest  InputSameDT=on
  Constant : Constant  DisableCoverage=on  Value=0  OutDataTypeStr=Inherit: Inherit via back propagation  PreserveConstantTs=on
  y : Outport
  wires:
  Constant/1 -> Compare/2
  u/1 -> Compare/1
  Compare/1 -> y/1

== system MATLAB_Function_lib/region_limit/Compare To Zero1 ==
  u : Inport
  Compare : RelationalOperator  Operator=<=  OutDataTypeStr=boolean  RndMeth=Nearest  InputSameDT=on
  Constant : Constant  DisableCoverage=on  Value=0  OutDataTypeStr=Inherit: Inherit via back propagation  PreserveConstantTs=on
  y : Outport
  wires:
  Constant/1 -> Compare/2
  u/1 -> Compare/1
  Compare/1 -> y/1

== system MATLAB_Function_lib/region_limit/Compare To Zero2 ==
  u : Inport
  Compare : RelationalOperator  Operator=>  OutDataTypeStr=boolean  RndMeth=Nearest  InputSameDT=on
  Constant : Constant  DisableCoverage=on  Value=0  OutDataTypeStr=Inherit: Inherit via back propagation  PreserveConstantTs=on
  y : Outport
  wires:
  Constant/1 -> Compare/2
  u/1 -> Compare/1
  Compare/1 -> y/1

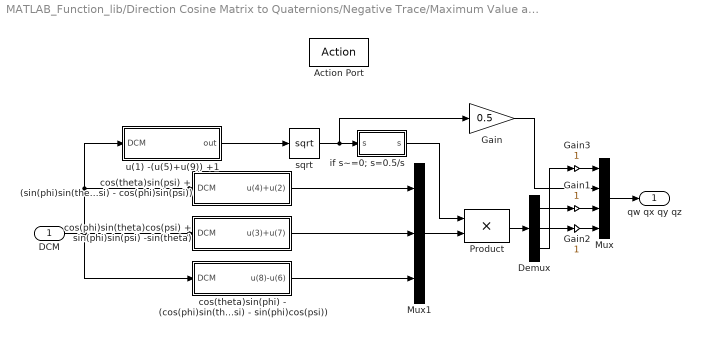
== system MATLAB_Function_lib/Direction Cosine Matrix to Quaternions/Negative Trace/Maximum Value at DCM(1,1) ==
  DCM : Inport
  Action Port : ActionPort  PropagateVarSize=During execution  ActionType=else
  Demux : Demux  Outputs=3
  Gain : Gain  Gain=0.5  SaturateOnIntegerOverflow=on  OutDataTypeStr=Inherit: Same as input  ParamDataTypeStr=Inherit: Same as input
  Gain1 : Gain  SaturateOnIntegerOverflow=on  OutDataTypeStr=Inherit: Same as input  ParamDataTypeStr=Inherit: Same as input
  Gain2 : Gain  SaturateOnIntegerOverflow=on  OutDataTypeStr=Inherit: Same as input  ParamDataTypeStr=Inherit: Same as input
  Gain3 : Gain  SaturateOnIntegerOverflow=on  OutDataTypeStr=Inherit: Same as input  ParamDataTypeStr=Inherit: Same as input
  Mux : Mux
  Mux1 : Mux  Inputs=3
  Product : Product  SaturateOnIntegerOverflow=on  InputSameDT=on  OutDataTypeStr=Inherit: Same as first input
  cos(phi)sin(theta)cos(psi) + sin(phi)sin(psi) -sin(theta) : Subsystem
  cos(theta)sin(phi) - (cos(phi)sin(theta)sin(psi) - sin(phi)cos(psi)) : Subsystem
  cos(theta)sin(psi) + (sin(phi)sin(theta)cos(psi) - cos(phi)sin(psi)) : Subsystem
  if s~=0; s=0.5/s : Subsystem
  sqrt : Sqrt  AlgorithmType=Newton-Raphson  SaturateOnIntegerOverflow=on
  u(1) -(u(5)+u(9)) +1 : Subsystem
  qw qx qy qz : Outport
  wires:
  u(1) -(u(5)+u(9)) +1/1(out) -> sqrt/1
  Gain1/1 -> Mux/3
  Gain/1 -> Mux/2
  if s~=0; s=0.5/s/1("s ") -> Product/1
  Product/1 -> Demux/1
  Demux/3 -> Gain3/1
  DCM/1 -> cos(phi)sin(theta)cos(psi) + sin(phi)sin(psi) -sin(theta)/1(DCM), cos(theta)sin(phi) - (cos(phi)sin(theta)sin(psi) - sin(phi)cos(psi))/1(DCM), cos(theta)sin(psi) + (sin(phi)sin(theta)cos(psi) - cos(phi)sin(psi))/1(DCM), u(1) -(u(5)+u(9)) +1/1(DCM)
  Gain3/1 -> Mux/1
  Gain2/1 -> Mux/4
  Mux/1 -> qw qx qy qz/1
  sqrt/1 -> if s~=0; s=0.5/s/1(s), Gain/1
  Mux1/1 -> Product/2
  cos(theta)sin(psi) + (sin(phi)sin(theta)cos(psi) - cos(phi)sin(psi))/1(u(4)+u(2)) -> Mux1/1
  cos(theta)sin(phi) - (cos(phi)sin(theta)sin(psi) - sin(phi)cos(psi))/1(u(8)-u(6)) -> Mux1/3
  Demux/2 -> Gain2/1
  cos(phi)sin(theta)cos(psi) + sin(phi)sin(psi) -sin(theta)/1(u(3)+u(7)) -> Mux1/2
  Demux/1 -> Gain1/1

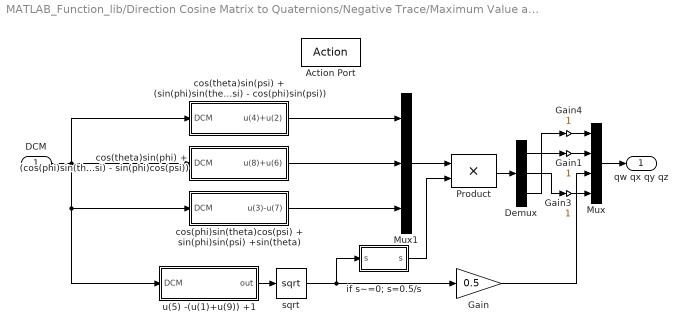
== system MATLAB_Function_lib/Direction Cosine Matrix to Quaternions/Negative Trace/Maximum Value at DCM(2,2) ==
  DCM : Inport
  Action Port : ActionPort  PropagateVarSize=During execution  ActionType=then
  Demux : Demux  Outputs=3
  Gain : Gain  Gain=0.5  SaturateOnIntegerOverflow=on  OutDataTypeStr=Inherit: Same as input  ParamDataTypeStr=Inherit: Same as input
  Gain1 : Gain  SaturateOnIntegerOverflow=on  OutDataTypeStr=Inherit: Same as input  ParamDataTypeStr=Inherit: Same as input
  Gain3 : Gain  SaturateOnIntegerOverflow=on  OutDataTypeStr=Inherit: Same as input  ParamDataTypeStr=Inherit: Same as input
  Gain4 : Gain  SaturateOnIntegerOverflow=on  OutDataTypeStr=Inherit: Same as input  ParamDataTypeStr=Inherit: Same as input
  Mux : Mux
  Mux1 : Mux  Inputs=3
  Product : Product  SaturateOnIntegerOverflow=on  InputSameDT=on  OutDataTypeStr=Inherit: Same as first input
  cos(phi)sin(theta)cos(psi) + sin(phi)sin(psi) +sin(theta) : Subsystem
  cos(theta)sin(phi) + (cos(phi)sin(theta)sin(psi) - sin(phi)cos(psi)) : Subsystem
  cos(theta)sin(psi) + (sin(phi)sin(theta)cos(psi) - cos(phi)sin(psi)) : Subsystem
  if s~=0; s=0.5/s : Subsystem
  sqrt : Sqrt  AlgorithmType=Newton-Raphson  SaturateOnIntegerOverflow=on
  u(5) -(u(1)+u(9)) +1 : Subsystem
  qw qx qy qz : Outport
  wires:
  u(5) -(u(1)+u(9)) +1/1(out) -> sqrt/1
  Demux/1 -> Gain1/1
  Demux/3 -> Gain4/1
  cos(theta)sin(psi) + (sin(phi)sin(theta)cos(psi) - cos(phi)sin(psi))/1(u(4)+u(2)) -> Mux1/1
  sqrt/1 -> Gain/1, if s~=0; s=0.5/s/1(s)
  Product/1 -> Demux/1
  Gain4/1 -> Mux/1
  Gain1/1 -> Mux/2
  cos(theta)sin(phi) + (cos(phi)sin(theta)sin(psi) - sin(phi)cos(psi))/1(u(8)+u(6)) -> Mux1/2
  Mux/1 -> qw qx qy qz/1
  cos(phi)sin(theta)cos(psi) + sin(phi)sin(psi) +sin(theta)/1(u(3)-u(7)) -> Mux1/3
  Demux/2 -> Gain3/1
  DCM/1 -> cos(theta)sin(phi) + (cos(phi)sin(theta)sin(psi) - sin(phi)cos(psi))/1(DCM), cos(theta)sin(psi) + (sin(phi)sin(theta)cos(psi) - cos(phi)sin(psi))/1(DCM), cos(phi)sin(theta)cos(psi) + sin(phi)sin(psi) +sin(theta)/1(DCM), u(5) -(u(1)+u(9)) +1/1(DCM)
  Gain/1 -> Mux/3
  if s~=0; s=0.5/s/1("s ") -> Product/2
  Mux1/1 -> Product/1
  Gain3/1 -> Mux/4

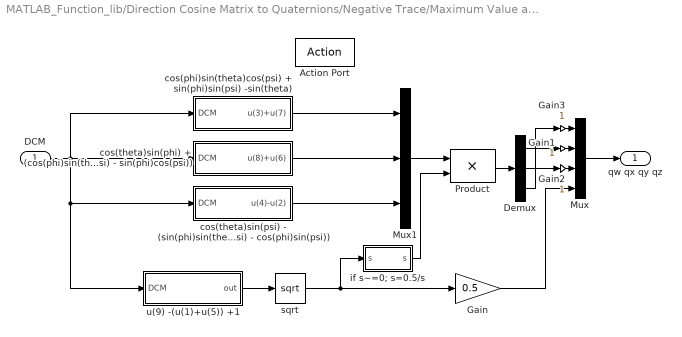
== system MATLAB_Function_lib/Direction Cosine Matrix to Quaternions/Negative Trace/Maximum Value at DCM(3,3) ==
  DCM : Inport
  Action Port : ActionPort  PropagateVarSize=During execution  ActionType=elseif
  Demux : Demux  Outputs=3
  Gain : Gain  Gain=0.5  SaturateOnIntegerOverflow=on  OutDataTypeStr=Inherit: Same as input  ParamDataTypeStr=Inherit: Same as input
  Gain1 : Gain  SaturateOnIntegerOverflow=on  OutDataTypeStr=Inherit: Same as input  ParamDataTypeStr=Inherit: Same as input
  Gain2 : Gain  SaturateOnIntegerOverflow=on  OutDataTypeStr=Inherit: Same as input  ParamDataTypeStr=Inherit: Same as input
  Gain3 : Gain  SaturateOnIntegerOverflow=on  OutDataTypeStr=Inherit: Same as input  ParamDataTypeStr=Inherit: Same as input
  Mux : Mux
  Mux1 : Mux  Inputs=3
  Product : Product  SaturateOnIntegerOverflow=on  InputSameDT=on  OutDataTypeStr=Inherit: Same as first input
  cos(phi)sin(theta)cos(psi) + sin(phi)sin(psi) -sin(theta) : Subsystem
  cos(theta)sin(phi) + (cos(phi)sin(theta)sin(psi) - sin(phi)cos(psi)) : Subsystem
  cos(theta)sin(psi) - (sin(phi)sin(theta)cos(psi) - cos(phi)sin(psi)) : Subsystem
  if s~=0; s=0.5/s : Subsystem
  sqrt : Sqrt  AlgorithmType=Newton-Raphson  SaturateOnIntegerOverflow=on
  u(9) -(u(1)+u(5)) +1 : Subsystem
  qw qx qy qz : Outport
  wires:
  Demux/3 -> Gain3/1
  Gain/1 -> Mux/4
  Demux/1 -> Gain1/1
  Product/1 -> Demux/1
  Gain1/1 -> Mux/2
  cos(theta)sin(phi) + (cos(phi)sin(theta)sin(psi) - sin(phi)cos(psi))/1(u(8)+u(6)) -> Mux1/2
  if s~=0; s=0.5/s/1("s ") -> Product/2
  cos(theta)sin(psi) - (sin(phi)sin(theta)cos(psi) - cos(phi)sin(psi))/1(u(4)-u(2)) -> Mux1/3
  Mux1/1 -> Product/1
  Demux/2 -> Gain2/1
  cos(phi)sin(theta)cos(psi) + sin(phi)sin(psi) -sin(theta)/1(u(3)+u(7)) -> Mux1/1
  Gain3/1 -> Mux/1
  DCM/1 -> cos(phi)sin(theta)cos(psi) + sin(phi)sin(psi) -sin(theta)/1(DCM), cos(theta)sin(phi) + (cos(phi)sin(theta)sin(psi) - sin(phi)cos(psi))/1(DCM), cos(theta)sin(psi) - (sin(phi)sin(theta)cos(psi) - cos(phi)sin(psi))/1(DCM), u(9) -(u(1)+u(5)) +1/1(DCM)
  sqrt/1 -> if s~=0; s=0.5/s/1(s), Gain/1
  u(9) -(u(1)+u(5)) +1/1(out) -> sqrt/1
  Mux/1 -> qw qx qy qz/1
  Gain2/1 -> Mux/3

== system MATLAB_Function_lib/Direction Cosine Matrix to Quaternions/Negative Trace/diag(DCM) ==
  DCM : Inport
  Demux : Demux  Outputs=3
  Selector : Selector  InputPortWidth=9  IndexOptions=Index vector (dialog)  Indices=[1 5 9]  OutputSizes=1
  u(1) : Outport
  u(5) : Outport  Port=2
  u(9) : Outport  Port=3
  wires:
  DCM/1 -> Selector/1
  Demux/3 -> u(9)/1
  Demux/2 -> u(5)/1
  Selector/1 -> Demux/1
  Demux/1 -> u(1)/1

== system MATLAB_Function_lib/Direction Cosine Matrix to Quaternions/Positive Trace/cos(phi)sin(theta)cos(psi) + sin(phi)sin(psi) +sin(theta) ==
  DCM : Inport
  Add : Sum  Inputs=+-|
  Demux : Demux  Outputs=2
  Selector : Selector  InputPortWidth=9  IndexOptions=Index vector (dialog)  Indices=[3 7]  OutputSizes=1
  u(3)-u(7) : Outport
  wires:
  Demux/1 -> Add/1
  Demux/2 -> Add/2
  Selector/1 -> Demux/1
  Add/1 -> u(3)-u(7)/1
  DCM/1 -> Selector/1

== system MATLAB_Function_lib/Direction Cosine Matrix to Quaternions/Positive Trace/cos(theta)sin(phi) - (cos(phi)sin(theta)sin(psi) - sin(phi)cos(psi)) ==
  DCM : Inport
  Add : Sum  Inputs=|-+
  Demux : Demux  Outputs=2
  Selector : Selector  InputPortWidth=9  IndexOptions=Index vector (dialog)  Indices=[6 8]  OutputSizes=1
  u(8)-u(6) : Outport
  wires:
  Add/1 -> u(8)-u(6)/1
  Demux/2 -> Add/2
  Demux/1 -> Add/1
  Selector/1 -> Demux/1
  DCM/1 -> Selector/1
